simulink model "untitled_F"  (R2013b)
settings: Solver=ode45  StartTime=0.0  StopTime=500  RelTol=1e-3
undefined symbols (not defined in the file): c, delta, ki, kp, Qs, R
settings Model: Creator=Yurii  LastModifiedBy=Yurii

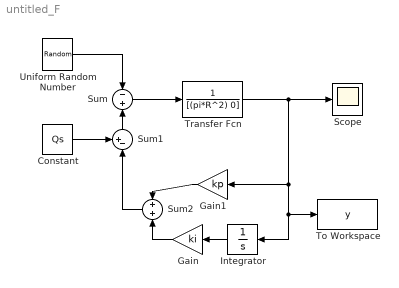
== system untitled_F ==
  Constant : Constant  Value=Qs
  Gain : Gain  Gain=ki
  Gain1 : Gain  Gain=kp
  Integrator : Integrator
  Scope : Scope
  Sum : Sum  Inputs=-|+
  Sum1 : Sum  Inputs=+-|
  Sum2 : Sum  Inputs=+|+
  To Workspace : ToWorkspace  VariableName=y  SampleTime=-1  SaveFormat=Timeseries
  Transfer Fcn : TransferFcn  Denominator=[(pi*R^2) 0]
  Uniform Random Number : UniformRandomNumber  Minimum=(c-delta)*Qs  Maximum=(c+delta)*Qs  SampleTime=0.1
  wires:
  Uniform Random Number/1 -> Sum/1
  Sum/1 -> Transfer Fcn/1
  Transfer Fcn/1 -> Gain1/1, To Workspace/1, Integrator/1, Scope/1
  Constant/1 -> Sum1/1
  Sum1/1 -> Sum/2
  Integrator/1 -> Gain/1
  Gain/1 -> Sum2/2
  Gain1/1 -> Sum2/1
  Sum2/1 -> Sum1/2
